simulink model "sslab_1"  (Simulink 10.1)
settings: Solver=ode45  StartTime=0.0  StopTime=10  RelTol=1e-3  EnableMultiTasking=on
values from neighbouring files (symbols this model uses):
  A = [1.4 -0.2 6.7 -5.7 ; -0.6 -4.3 0 0.7 ; 1.1 4.3 -6.7 5.9 ... (first row only)    [main.m]    (also in sslabsc.m = Ao)
  Ao = [1.38 -0.2077 6.715 -5.676 ... (first row only)    [sslabsc.m]
  B = [ 0 0 ; 5.7 0 ; 1.1 -3.1 ; 1.1 0 ]    [main.m]    (also in sslabsc.m = Bo)
  Bo = [0 0; 5.679 0; 1.136 -3.146; 1.136 0]    [sslabsc.m]
  C = [1 0 0 0 ; 0 1 0 0 ; 0 0 1 -1]    [main.m]    (also in sslabsc.m = Co)
  Co = [1 0 0 0; 0 1 0 0; 0 0 1 -1]    [sslabsc.m]
  D = [0 0 ; 0 0 ; 0 0]    [main.m]    (also in sslabsc.m = Do)
  Do = zeros(3,2)    [sslabsc.m]
  Kaug = K_aug(:,1:4)    [main.m]
  Ki = -K_aug(:,5:end)    [main.m]
  kr = k_u + K_2*k_x    [main.m]    (also in sslabsc.m = [1 0; 0 1])
  L1 = K4'    [main.m]
libraries: simulink x1
settings Model: Creator=bjones  LastModifiedBy=ACER  ExtModeTrigMode=oneshot  ExtModeArmWhenConnect=off
settings DataIOCC: SignalLoggingSaveFormat=ModelDataLogs
settings OptimizationCC: BlockReduction=off  BooleanDataType=off  ExpressionDepthLimit=2147483647  InitFltsAndDblsToZero=on
settings DebuggingCC: SaveWithParameterizedLinksMsg=none  SignalResolutionControl=TryResolveAllWithWarning  MultiTaskDSMMsg=warning  MultiTaskCondExecSysMsg=none  FcnCallInpInsideContextMsg=warning  StateNameClashWarn=warning
settings HardwareCC: TargetUnknown=on
settings GRTTargetCC: TargetFcnLib=ansi_tfl_tmw.mat  ModelReferenceCompliant=off  ParMdlRefBuildCompliant=off  CompOptLevelCompliant=off  MatFileLogging=off

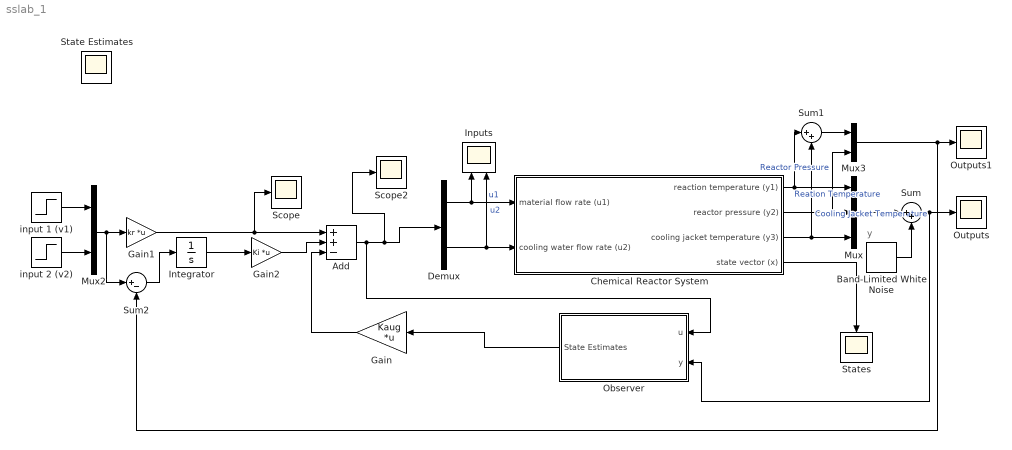
== system sslab_1 ==
  note: y
  Add : Sum  Inputs=++-
  Band-Limited White Noise : simulink/Sources/Band-Limited White Noise  Cov=1e-5  Ts=0.1  seed=[23341]
  Chemical Reactor System : Subsystem  mask(System Block){}
      mask help: Chemical reactor system used for the ACS6129 laboratory. Please ask a demonstrator or press help if you are interested in the underlying workings of the system.
      mask Help:
      | This is the chemical reactor system block for use in the ACS6129 laboratory. This block implements a continuous time state space model of the system, using a set of pre-defined system matrices found in the sslabsc.m file.
      | 
      | This block should not be edited, and for further information about the block please ask a demonstrator.
  Demux : Demux  Outputs=2
  Gain : Gain  Gain=Kaug  Multiplication=Matrix(K*u)
  Gain1 : Gain  Gain=kr  Multiplication=Matrix(K*u)
  Gain2 : Gain  Gain=Ki  Multiplication=Matrix(K*u)
  Inputs : Scope  NumInputPorts=2
  Integrator : Integrator
  Mux : Mux  Inputs=3
  Mux2 : Mux  Inputs=2
  Mux3 : Mux  Inputs=2
  Observer : Subsystem
  Outputs : Scope
  Outputs1 : Scope
  Scope : Scope
  Scope2 : Scope
  State Estimates : Scope
  States : Scope
  Sum : Sum  Inputs=|++
  Sum1 : Sum  Inputs=|++
  Sum2 : Sum  Inputs=|+-
  input 1 (v1) : Step  SampleTime=0
  input 2 (v2) : Step  SampleTime=0
  wires:
  input 1 (v1)/1 -> Mux2/1
  input 2 (v2)/1 -> Mux2/2
  Chemical Reactor System/1(reaction temperature (y1)) -> Sum1/1, Mux/1  "Reation Temperature"
  Chemical Reactor System/2(reactor pressure (y2)) -> Mux3/2, Mux/2  "Reactor Pressure"
  Chemical Reactor System/3(cooling jacket temperature (y3)) -> Mux/3, Sum1/2  "Cooling Jacket Temperature"
  Demux/1 -> Chemical Reactor System/1(material flow rate (u1)), Inputs/1  "u1"
  Demux/2 -> Chemical Reactor System/2(cooling water flow rate (u2)), Inputs/2  "u2"
  Add/1 -> Observer/1(u), Scope2/1, Demux/1
  Sum1/1 -> Mux3/1
  Mux3/1 -> Sum2/2, Outputs1/1
  Gain2/1 -> Add/2
  Integrator/1 -> Gain2/1
  Sum2/1 -> Integrator/1
  Mux2/1 -> Gain1/1, Sum2/1
  Chemical Reactor System/4(state vector (x)) -> States/1
  Gain/1 -> Add/3
  Gain1/1 -> Scope/1, Add/1
  Observer/1(State Estimates) -> Gain/1
  Mux/1 -> Sum/1
  Band-Limited White Noise/1 -> Sum/2
  Sum/1 -> Observer/2(y), Outputs/1

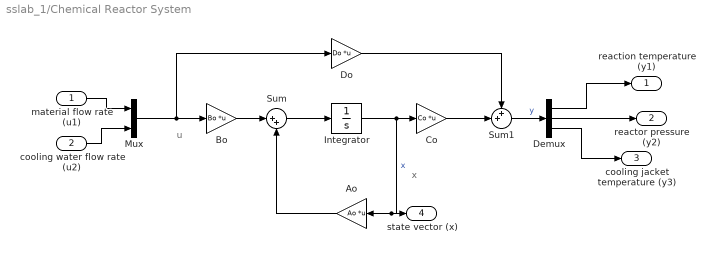
== system sslab_1/Chemical Reactor System ==
  note: u
  note: x
  material flow rate (u1) : Inport
  cooling water flow rate (u2) : Inport  Port=2
  Ao : Gain  Gain=Ao  Multiplication=Matrix(K*u)  SaturateOnIntegerOverflow=on  OutDataTypeStr=Inherit: Same as input  ParamDataTypeStr=Inherit: Same as input
  Bo : Gain  Gain=Bo  Multiplication=Matrix(K*u)  SaturateOnIntegerOverflow=on  OutDataTypeStr=Inherit: Same as input  ParamDataTypeStr=Inherit: Same as input
  Co : Gain  Gain=Co  Multiplication=Matrix(K*u)  SaturateOnIntegerOverflow=on  OutDataTypeStr=Inherit: Same as input  ParamDataTypeStr=Inherit: Same as input
  Demux : Demux  Outputs=3
  Do : Gain  Gain=Do  Multiplication=Matrix(K*u)  SaturateOnIntegerOverflow=on  OutDataTypeStr=Inherit: Same as input  ParamDataTypeStr=Inherit: Same as input
  Integrator : Integrator
  Mux : Mux  Inputs=2
  Sum : Sum  Inputs=|++  InputSameDT=on  SaturateOnIntegerOverflow=on  OutDataTypeStr=Inherit: Same as first input
  Sum1 : Sum  Inputs=++|  InputSameDT=on  SaturateOnIntegerOverflow=on  OutDataTypeStr=Inherit: Same as first input
  reaction temperature (y1) : Outport
  reactor pressure (y2) : Outport  Port=2
  cooling jacket temperature (y3) : Outport  Port=3
  state vector (x) : Outport  Port=4
  wires:
  Integrator/1 -> Co/1, Ao/1, state vector (x)/1  "x"
  Sum/1 -> Integrator/1
  Bo/1 -> Sum/1
  Ao/1 -> Sum/2
  Do/1 -> Sum1/1
  Co/1 -> Sum1/2
  Mux/1 -> Bo/1, Do/1
  material flow rate (u1)/1 -> Mux/1
  cooling water flow rate (u2)/1 -> Mux/2
  Sum1/1 -> Demux/1  "y"
  Demux/1 -> reaction temperature (y1)/1
  Demux/2 -> reactor pressure (y2)/1
  Demux/3 -> cooling jacket temperature (y3)/1

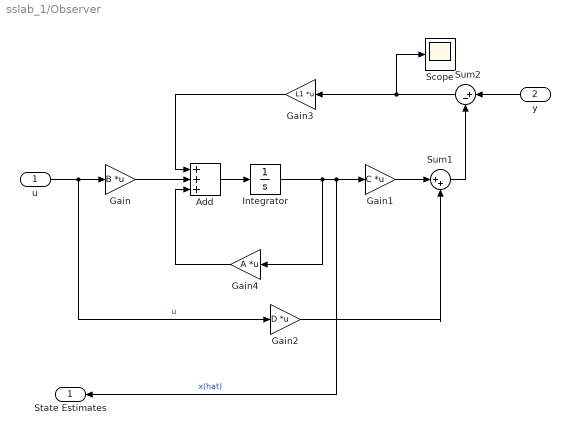
== system sslab_1/Observer ==
  u : Inport
  y : Inport  Port=2
  Add : Sum  Inputs=+++
  Gain : Gain  Gain=B  Multiplication=Matrix(K*u)
  Gain1 : Gain  Gain=C  Multiplication=Matrix(K*u)
  Gain2 : Gain  Gain=D  Multiplication=Matrix(K*u)
  Gain3 : Gain  Gain=L1  Multiplication=Matrix(K*u)
  Gain4 : Gain  Gain=A  Multiplication=Matrix(K*u)
  Integrator : Integrator  InitialCondition=[1 -1 0.5 -0.5]'
  Scope : Scope
  Sum1 : Sum  Inputs=|++
  Sum2 : Sum  Inputs=|+-
  State Estimates : Outport
  wires:
  u/1 -> Gain/1, Gain2/1  "u"
  y/1 -> Sum2/1
  Integrator/1 -> Gain4/1, State Estimates/1, Gain1/1  "x(hat)"
  Gain1/1 -> Sum1/1
  Gain2/1 -> Sum1/2
  Sum1/1 -> Sum2/2
  Sum2/1 -> Scope/1, Gain3/1
  Gain/1 -> Add/2
  Add/1 -> Integrator/1
  Gain3/1 -> Add/1
  Gain4/1 -> Add/3
